simulink model "MME321_Lab6_Simscape"  (R2024a)
settings: Solver=VariableStepAuto  StartTime=0.0  StopTime=1  MaxStep=0.001  RelTol=1e-3
libraries: fl_lib x70, nesl_utility x21, ee_lib x2
settings Model: Creator=buttrakd  LastModifiedBy=buttrakd

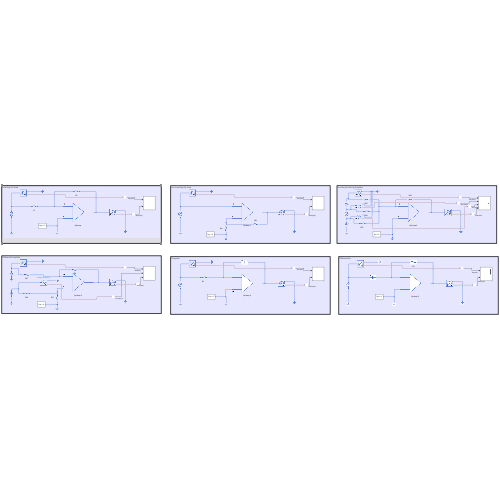
[thumbnail: Simulink's stored preview of the top-level diagram]
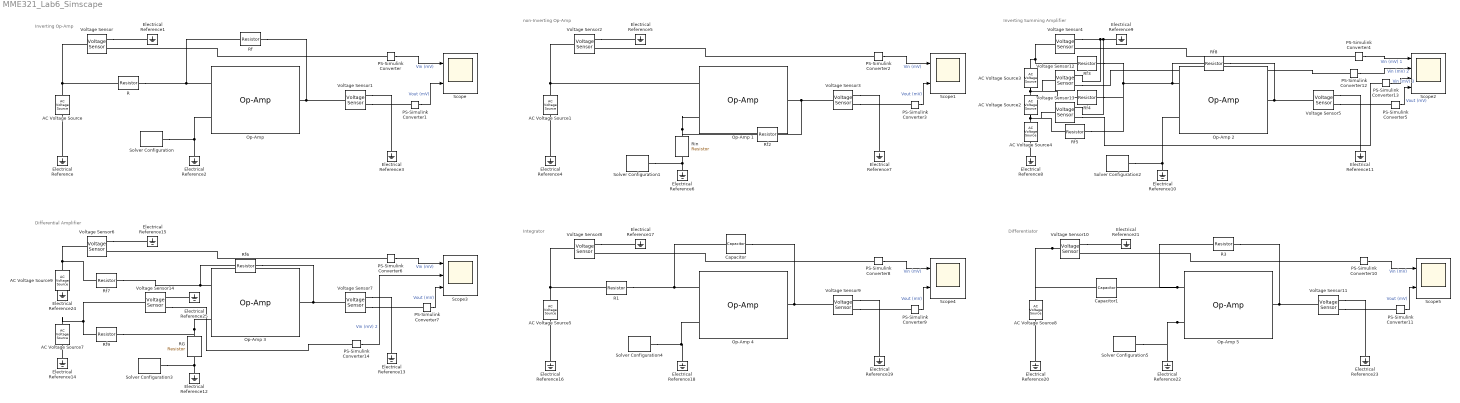
== system MME321_Lab6_Simscape ==
  note: Inverting Op-Amp
  note: non-Inverting Op-Amp
  note: Inverting Summing Amplifier
  note: Differential Amplifier
  note: Integrator
  note: Differentiator
  AC Voltage Source : fl_lib/Electrical/Electrical Sources/AC Voltage Source  amp=1 mV  shift=0 deg  frequency=5 Hz
  AC Voltage Source1 : fl_lib/Electrical/Electrical Sources/AC Voltage Source  amp=1 mV  shift=0 deg  frequency=5 Hz
  AC Voltage Source2 : fl_lib/Electrical/Electrical Sources/AC Voltage Source  amp=10 mV  shift=0 deg  frequency=5 Hz
  AC Voltage Source3 : fl_lib/Electrical/Electrical Sources/AC Voltage Source  amp=15 mV  shift=0 deg  frequency=5 Hz
  AC Voltage Source4 : fl_lib/Electrical/Electrical Sources/AC Voltage Source  amp=5 mV  shift=0 deg  frequency=5 Hz
  AC Voltage Source5 : fl_lib/Electrical/Electrical Sources/AC Voltage Source  amp=10 mV  shift=0 deg  frequency=5 Hz
  AC Voltage Source7 : fl_lib/Electrical/Electrical Sources/AC Voltage Source  amp=5 mV  shift=0 deg  frequency=5 Hz
  AC Voltage Source8 : fl_lib/Electrical/Electrical Sources/AC Voltage Source  amp=10 mV  shift=0 deg  frequency=5 Hz
  AC Voltage Source9 : fl_lib/Electrical/Electrical Sources/AC Voltage Source  amp=15 mV  shift=0 deg  frequency=5 Hz
  Capacitor : ee_lib/Passive/Capacitor  cap_option=ee.enum.passive.capacitor.capOption.const  c=1 uF  Cvec=[1e-05, 1e-06] F  Vvec=[0, 10] V  CV_table_symmetry=ee.enum.passive.capacitor.tableSymmetry.yes  f_vec=[1, 10] kHz  DFext_vec=[.8, 1.2]  enable_C_tol=ee.enum.toleranceApplication.none  averaging_period=0 s  C_tol=5  tol_distribution=ee.enum.toleranceDistribution.uniform  nSigma=4  r=0 Ohm  g=0 1/Ohm  maxPermissibleTemperature=85 degC  tFailOnTemperature=1 s  enable_operating_limits=ee.enum.enable.no  operating_limit_action=ee.enum.passive.reportOpLim.warn  max_working_voltage_range=[-25, 25] V  power_rating=1 W  maxTemperature=85 degC  thermalEnable=false  thermalMass=1 J/K  enable_faults=ee.enum.enable.no  fault_action=simscape.enum.assert.action.none  Cscale_faulted=100  R_faulted=1e-3 Ohm  G_faulted=0 1/Ohm  tau_fault=1e-3 s  fault_trigger=ee.enum.faults.faultTrigger.temporal  t_fault=1 s  max_permissible_voltage_range=[-100, 100] V  t_fail_on_voltage=1 s  i_specify=off  i_priority=None  i=0 A  i_nominal_specify=off  i_nominal_value=1  i_nominal_unit=A  v_specify=off  v_priority=None  v=0 V  v_nominal_specify=off  v_nominal_value=1  v_nominal_unit=V  vc_specify=off  vc_priority=High  vc=0 V  vc_nominal_specify=off  vc_nominal_value=1  vc_nominal_unit=V  T_specify=off  T_priority=None  T=298.15 K  T_nominal_specify=off  T_nominal_value=1  T_nominal_unit=K
  Capacitor1 : ee_lib/Passive/Capacitor  cap_option=ee.enum.passive.capacitor.capOption.const  c=1 uF  Cvec=[1e-05, 1e-06] F  Vvec=[0, 10] V  CV_table_symmetry=ee.enum.passive.capacitor.tableSymmetry.yes  f_vec=[1, 10] kHz  DFext_vec=[.8, 1.2]  enable_C_tol=ee.enum.toleranceApplication.none  averaging_period=0 s  C_tol=5  tol_distribution=ee.enum.toleranceDistribution.uniform  nSigma=4  r=0 Ohm  g=0 1/Ohm  maxPermissibleTemperature=85 degC  tFailOnTemperature=1 s  enable_operating_limits=ee.enum.enable.no  operating_limit_action=ee.enum.passive.reportOpLim.warn  max_working_voltage_range=[-25, 25] V  power_rating=1 W  maxTemperature=85 degC  thermalEnable=false  thermalMass=1 J/K  enable_faults=ee.enum.enable.no  fault_action=simscape.enum.assert.action.none  Cscale_faulted=100  R_faulted=1e-3 Ohm  G_faulted=0 1/Ohm  tau_fault=1e-3 s  fault_trigger=ee.enum.faults.faultTrigger.temporal  t_fault=1 s  max_permissible_voltage_range=[-100, 100] V  t_fail_on_voltage=1 s  i_specify=off  i_priority=None  i=0 A  i_nominal_specify=off  i_nominal_value=1  i_nominal_unit=A  v_specify=off  v_priority=None  v=0 V  v_nominal_specify=off  v_nominal_value=1  v_nominal_unit=V  vc_specify=off  vc_priority=High  vc=0 V  vc_nominal_specify=off  vc_nominal_value=1  vc_nominal_unit=V  T_specify=off  T_priority=None  T=298.15 K  T_nominal_specify=off  T_nominal_value=1  T_nominal_unit=K
  Electrical Reference{,1..25} (26 alike) : fl_lib/Electrical/Electrical Elements/Electrical Reference
  Op-Amp {,1..5} (6 alike) : fl_lib/Electrical/Electrical Elements/Op-Amp  outI_specify=off  outI_priority=None  outI=0 A  outI_nominal_specify=off  outI_nominal_value=1  outI_nominal_unit=A
  PS-Simulink Converter{,1..14} (15 alike) : nesl_utility/PS-Simulink Converter  PhysicalDomain=network_engine_domain  SubClassName=ps_output  LeftPortType=input  RightPortType=output  PseudoPeriodic=off  Frequencies=[]  VectorFormat=inherit  Unit=inherit  AffineConversion=off
  R : fl_lib/Electrical/Electrical Elements/Resistor  R=1 Ohm  i_specify=off  i_priority=None  i=0 A  i_nominal_specify=off  i_nominal_value=1  i_nominal_unit=A  v_specify=off  v_priority=None  v=0 V  v_nominal_specify=off  v_nominal_value=1  v_nominal_unit=V
  R1 : fl_lib/Electrical/Electrical Elements/Resistor  R=318 kOhm  i_specify=off  i_priority=None  i=0 A  i_nominal_specify=off  i_nominal_value=1  i_nominal_unit=A  v_specify=off  v_priority=None  v=0 V  v_nominal_specify=off  v_nominal_value=1  v_nominal_unit=V
  R3 : fl_lib/Electrical/Electrical Elements/Resistor  R=318 kOhm  i_specify=off  i_priority=None  i=0 A  i_nominal_specify=off  i_nominal_value=1  i_nominal_unit=A  v_specify=off  v_priority=None  v=0 V  v_nominal_specify=off  v_nominal_value=1  v_nominal_unit=V
  RG : fl_lib/Electrical/Electrical Elements/Resistor  R=10 Ohm  i_specify=off  i_priority=None  i=0 A  i_nominal_specify=off  i_nominal_value=1  i_nominal_unit=A  v_specify=off  v_priority=None  v=0 V  v_nominal_specify=off  v_nominal_value=1  v_nominal_unit=V
  Rf : fl_lib/Electrical/Electrical Elements/Resistor  R=10 Ohm  i_specify=off  i_priority=None  i=0 A  i_nominal_specify=off  i_nominal_value=1  i_nominal_unit=A  v_specify=off  v_priority=None  v=0 V  v_nominal_specify=off  v_nominal_value=1  v_nominal_unit=V
  Rf2 : fl_lib/Electrical/Electrical Elements/Resistor  R=9 Ohm  i_specify=off  i_priority=None  i=0 A  i_nominal_specify=off  i_nominal_value=1  i_nominal_unit=A  v_specify=off  v_priority=None  v=0 V  v_nominal_specify=off  v_nominal_value=1  v_nominal_unit=V
  Rf{3..5,7,9} (5 alike) : fl_lib/Electrical/Electrical Elements/Resistor  R=1 Ohm  i_specify=off  i_priority=None  i=0 A  i_nominal_specify=off  i_nominal_value=1  i_nominal_unit=A  v_specify=off  v_priority=None  v=0 V  v_nominal_specify=off  v_nominal_value=1  v_nominal_unit=V
  Rf6 : fl_lib/Electrical/Electrical Elements/Resistor  R=10 Ohm  i_specify=off  i_priority=None  i=0 A  i_nominal_specify=off  i_nominal_value=1  i_nominal_unit=A  v_specify=off  v_priority=None  v=0 V  v_nominal_specify=off  v_nominal_value=1  v_nominal_unit=V
  Rf8 : fl_lib/Electrical/Electrical Elements/Resistor  R=10 Ohm  i_specify=off  i_priority=None  i=0 A  i_nominal_specify=off  i_nominal_value=1  i_nominal_unit=A  v_specify=off  v_priority=None  v=0 V  v_nominal_specify=off  v_nominal_value=1  v_nominal_unit=V
  Rin : fl_lib/Electrical/Electrical Elements/Resistor  R=1 Ohm  i_specify=off  i_priority=None  i=0 A  i_nominal_specify=off  i_nominal_value=1  i_nominal_unit=A  v_specify=off  v_priority=None  v=0 V  v_nominal_specify=off  v_nominal_value=1  v_nominal_unit=V
  Scope{,1,4..5} (4 alike) : Scope  NumInputPorts=2
  Scope2 : Scope  NumInputPorts=4
  Scope3 : Scope  NumInputPorts=3
  Solver Configuration{,1..5} (6 alike) : nesl_utility/Solver Configuration  PhysicalDomain=network_engine_domain  SubClassName=solver  LeftPortType=input  RightPortType=generic  Tones=[]  Harmonics=[]  SimulateNoise=off  Profile=off  UseLocalSampling=off  EnableSwitchedLinearOptims=on  FrequencyDomain=off  UseCCode=off  RelTol=0.001  AbsTol=0.001  MinStep=1e-09  ToWorkspace=off  RevertToSquareIcSolve=off  NumHomotopyIterations=100  PhasorMode=off  PhasorModeNumHarmonics=1  ConsistencySolver=NEWTON_XTOL_AFTER_FTOL  IndexReductionMethod=DerivativeReplacement  DoDC=off  ResidualTolerance=1e-09  ConsistencyTolSource=GLOBAL  ConsistencyAbsTol=0.001  ConsistencyRelTol=0.001  ConsistencyTolFactor=0.001  UseLocalSolver=off  LocalSolverChoice=NE_BACKWARD_EULER_ADVANCER  ResolveIndetEquations=on  FunctionEvalNumThread=1  LocalSolverSampleTime=0.001  DoFixedCost=off  MaxNonlinIter=3  MaxModeIter=2  ComputeImpulses=off  ImpulseIterations=2  LinearAlgebra=auto  LinearAlgebraNumThread=0  EquationFormulation=NE_TIME_EF  DelaysMemoryBudget=1024  AutomaticFiltering=on  FilteringTimeConstant=0.001  PartitionStorageMethod=AS_NEEDED  PartitionMemoryBudget=1024  PartitionMethod=ROBUST  MultibodyUseLocalSolver=off  MultibodyLocalSolverChoice=ODE1  MultibodyLocalSolverSampleTime=0.001
  Voltage Sensor{,1..14} (15 alike) : fl_lib/Electrical/Electrical Sensors/Voltage Sensor
  wires:
  PS-Simulink Converter1/1 -> Scope/2  "Vout (mV)"
  PS-Simulink Converter/1 -> Scope/1  "Vin (mV)"
  PS-Simulink Converter2/1 -> Scope1/1  "Vin (mV)"
  PS-Simulink Converter3/1 -> Scope1/2  "Vout (mV)"
  PS-Simulink Converter5/1 -> Scope2/4  "Vout (mV)"
  PS-Simulink Converter4/1 -> Scope2/1  "Vin (mV) 1"
  PS-Simulink Converter6/1 -> Scope3/1  "Vin (mV)"
  PS-Simulink Converter7/1 -> Scope3/3  "Vout (mV)"
  PS-Simulink Converter8/1 -> Scope4/1  "Vin (mV)"
  PS-Simulink Converter9/1 -> Scope4/2  "Vout (mV)"
  PS-Simulink Converter11/1 -> Scope5/2  "Vout (mV)"
  PS-Simulink Converter10/1 -> Scope5/1  "Vin (mV)"
  PS-Simulink Converter12/1 -> Scope2/2  "Vin (mV) 2"
  PS-Simulink Converter13/1 -> Scope2/3  "Vin (mV) 3"
  PS-Simulink Converter14/1 -> Scope3/2  "Vin (mV) 2"
  connections:
  Voltage Sensor/RConn2 -- Electrical Reference1/LConn1
  AC Voltage Source/LConn1 -- R/LConn1 -- Voltage Sensor/LConn1
  Electrical Reference/LConn1 -- AC Voltage Source/RConn1
  R/RConn1 -- Rf/LConn1 -- "Op-Amp "/LConn1
  Electrical Reference2/LConn1 -- Solver Configuration/RConn1 -- "Op-Amp "/LConn2
  Voltage Sensor1/LConn1 -- Rf/RConn1 -- "Op-Amp "/RConn1
  Voltage Sensor1/RConn2 -- Electrical Reference3/LConn1
  Voltage Sensor1/RConn1 -- PS-Simulink Converter1/LConn1
  PS-Simulink Converter/LConn1 -- Voltage Sensor/RConn1
  AC Voltage Source1/LConn1 -- Op-Amp 1/LConn1 -- Voltage Sensor2/LConn1
  Rin/LConn1 -- Rf2/RConn1 -- Op-Amp 1/LConn2
  Voltage Sensor3/LConn1 -- Rf2/LConn1 -- Op-Amp 1/RConn1
  PS-Simulink Converter2/LConn1 -- Voltage Sensor2/RConn1
  Voltage Sensor3/RConn1 -- PS-Simulink Converter3/LConn1
  Voltage Sensor3/RConn2 -- Electrical Reference7/LConn1
  Electrical Reference4/LConn1 -- AC Voltage Source1/RConn1
  Voltage Sensor2/RConn2 -- Electrical Reference5/LConn1
  Solver Configuration1/RConn1 -- Rin/RConn1 -- Electrical Reference6/LConn1
  Solver Configuration2/RConn1 -- Op-Amp 2/LConn2 -- Electrical Reference10/LConn1
  Op-Amp 2/RConn1 -- Rf8/LConn1 -- Voltage Sensor5/LConn1
  Electrical Reference8/LConn1 -- AC Voltage Source4/RConn1
  Voltage Sensor4/RConn2 -- Voltage Sensor12/RConn2 -- Electrical Reference9/LConn1 -- Voltage Sensor13/RConn2
  Voltage Sensor5/RConn2 -- Electrical Reference11/LConn1
  Voltage Sensor5/RConn1 -- PS-Simulink Converter5/LConn1
  PS-Simulink Converter4/LConn1 -- Voltage Sensor4/RConn1
  Rf3/LConn1 -- Voltage Sensor4/LConn1 -- AC Voltage Source3/LConn1
  AC Voltage Source2/LConn1 -- Voltage Sensor12/LConn1 -- Rf4/LConn1 -- AC Voltage Source3/RConn1
  AC Voltage Source4/LConn1 -- Voltage Sensor13/LConn1 -- Rf5/LConn1 -- AC Voltage Source2/RConn1
  Rf5/RConn1 -- Rf4/RConn1 -- Rf3/RConn1 -- Rf8/RConn1 -- Op-Amp 2/LConn1
  RG/LConn1 -- Op-Amp 3/LConn2 -- Rf9/RConn1
  Rf6/RConn1 -- Op-Amp 3/RConn1 -- Voltage Sensor7/LConn1
  Rf7/LConn1 -- AC Voltage Source9/RConn1 -- Voltage Sensor6/LConn1
  AC Voltage Source7/LConn1 -- Rf9/LConn1 -- Voltage Sensor14/LConn1
  Rf7/RConn1 -- Op-Amp 3/LConn1 -- Rf6/LConn1
  Voltage Sensor7/RConn2 -- Electrical Reference13/LConn1
  Voltage Sensor7/RConn1 -- PS-Simulink Converter7/LConn1
  Voltage Sensor6/RConn2 -- Electrical Reference15/LConn1
  PS-Simulink Converter6/LConn1 -- Voltage Sensor6/RConn1
  Electrical Reference14/LConn1 -- AC Voltage Source7/RConn1
  Electrical Reference12/LConn1 -- Solver Configuration3/RConn1 -- RG/RConn1
  AC Voltage Source5/LConn1 -- Voltage Sensor8/LConn1 -- R1/LConn1
  R1/RConn1 -- Op-Amp 4/LConn2 -- Capacitor/LConn1
  Solver Configuration4/RConn1 -- Op-Amp 4/LConn1 -- Electrical Reference18/LConn1
  Op-Amp 4/RConn1 -- Capacitor/RConn1 -- Voltage Sensor9/LConn1
  PS-Simulink Converter8/LConn1 -- Voltage Sensor8/RConn1
  Voltage Sensor9/RConn1 -- PS-Simulink Converter9/LConn1
  Voltage Sensor9/RConn2 -- Electrical Reference19/LConn1
  Electrical Reference16/LConn1 -- AC Voltage Source5/RConn1
  Voltage Sensor8/RConn2 -- Electrical Reference17/LConn1
  Voltage Sensor10/LConn1 -- Capacitor1/LConn1 -- AC Voltage Source8/LConn1
  Op-Amp 5/LConn1 -- Capacitor1/RConn1 -- R3/LConn1
  Op-Amp 5/LConn2 -- Electrical Reference22/LConn1 -- Solver Configuration5/RConn1
  Voltage Sensor11/LConn1 -- R3/RConn1 -- Op-Amp 5/RConn1
  Voltage Sensor11/RConn2 -- Electrical Reference23/LConn1
  Voltage Sensor11/RConn1 -- PS-Simulink Converter11/LConn1
  PS-Simulink Converter10/LConn1 -- Voltage Sensor10/RConn1
  Voltage Sensor10/RConn2 -- Electrical Reference21/LConn1
  Electrical Reference20/LConn1 -- AC Voltage Source8/RConn1
  Voltage Sensor12/RConn1 -- PS-Simulink Converter12/LConn1
  Voltage Sensor13/RConn1 -- PS-Simulink Converter13/LConn1
  Electrical Reference24/LConn1 -- AC Voltage Source9/LConn1
  Voltage Sensor14/RConn1 -- PS-Simulink Converter14/LConn1
  Electrical Reference25/LConn1 -- Voltage Sensor14/RConn2
